simulink model "svpwm_inv_Motor_new_sent"  (R2022b)
settings: Solver=daessc  StartTime=0.0  StopTime=0.62  MaxStep=2.5e-6  RelTol=1e-3
libraries: nesl_utility x37, fl_lib x34, ee_lib x21, spsMeanLib x9, simulink x6, slpidlib x4, mcbcontrolslib x3, simulink_extras x1
(part 2 of 2)

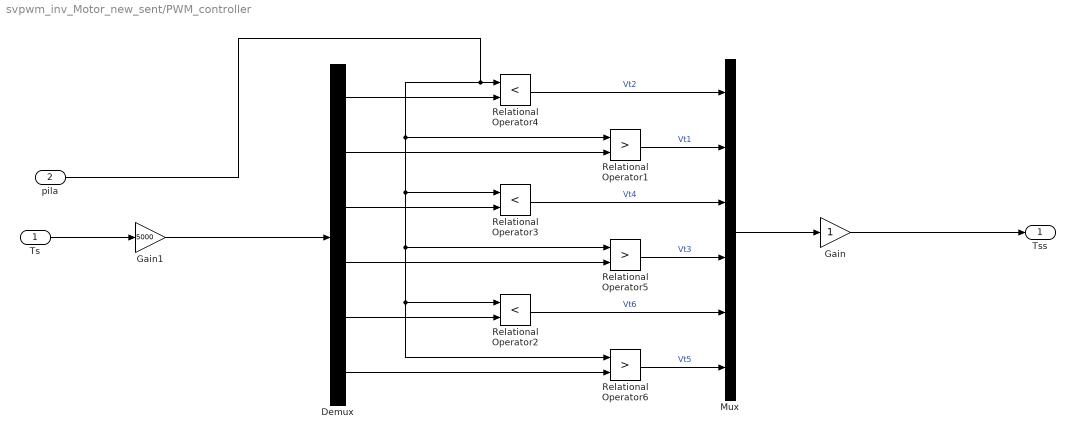
== system svpwm_inv_Motor_new_sent/PWM_controller ==
  Ts : Inport
  pila : Inport  Port=2
  Demux : Demux  Outputs=6
  Gain : Gain  ParamDataTypeStr=double
  Gain1 : Gain  Gain=5000
  Mux : Mux  Inputs=6
  Relational Operator1 : RelationalOperator  Operator=>  OutDataTypeStr=boolean  InputSameDT=off
  Relational Operator2 : RelationalOperator  Operator=<  OutDataTypeStr=boolean  InputSameDT=off
  Relational Operator3 : RelationalOperator  Operator=<  OutDataTypeStr=boolean  InputSameDT=off
  Relational Operator4 : RelationalOperator  Operator=<  OutDataTypeStr=boolean  InputSameDT=off
  Relational Operator5 : RelationalOperator  Operator=>  OutDataTypeStr=boolean  InputSameDT=off
  Relational Operator6 : RelationalOperator  Operator=>  OutDataTypeStr=boolean  InputSameDT=off
  Tss : Outport  VectorParamsAs1DForOutWhenUnconnected=off
  wires:
  Relational Operator4/1 -> Mux/1  "Vt2"
  Demux/3 -> Relational Operator3/2
  Demux/5 -> Relational Operator2/2
  Relational Operator3/1 -> Mux/3  "Vt4"
  Relational Operator2/1 -> Mux/5  "Vt6"
  Ts/1 -> Gain1/1
  pila/1 -> Relational Operator1/1, Relational Operator3/1, Relational Operator5/1, Relational Operator2/1, Relational Operator6/1, Relational Operator4/1
  Relational Operator1/1 -> Mux/2  "Vt1"
  Relational Operator5/1 -> Mux/4  "Vt3"
  Relational Operator6/1 -> Mux/6  "Vt5"
  Demux/2 -> Relational Operator1/2
  Demux/4 -> Relational Operator5/2
  Demux/6 -> Relational Operator6/2
  Demux/1 -> Relational Operator4/2
  Mux/1 -> Gain/1
  Gain/1 -> Tss/1
  Gain1/1 -> Demux/1

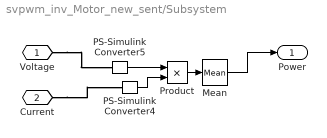
== system svpwm_inv_Motor_new_sent/Subsystem ==
  Mean : spsMeanLib/Mean  Freq=5000  Vinit=0  Ts=0
  PS-Simulink Converter4 : nesl_utility/PS-Simulink Converter  PhysicalDomain=network_engine_domain  SubClassName=ps_output  LeftPortType=input  RightPortType=output  PseudoPeriodic=off  Frequencies=[]  VectorFormat=inherit  Unit=inherit  AffineConversion=off
  PS-Simulink Converter5 : nesl_utility/PS-Simulink Converter  PhysicalDomain=network_engine_domain  SubClassName=ps_output  LeftPortType=input  RightPortType=output  PseudoPeriodic=off  Frequencies=[]  VectorFormat=inherit  Unit=inherit  AffineConversion=off
  Product : Product
  Voltage : PMIOPort  Side=Left
  Current : PMIOPort  Port=2  Side=Left
  Power : Outport
  wires:
  Product/1 -> Mean/1
  PS-Simulink Converter5/1 -> Product/1
  PS-Simulink Converter4/1 -> Product/2
  Mean/1 -> Power/1
  connections:
  Current/RConn1 -- PS-Simulink Converter4/LConn1
  Voltage/RConn1 -- PS-Simulink Converter5/LConn1

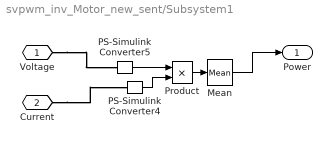
== system svpwm_inv_Motor_new_sent/Subsystem1 ==
  Mean : spsMeanLib/Mean  Freq=5000  Vinit=0  Ts=0
  PS-Simulink Converter4 : nesl_utility/PS-Simulink Converter  PhysicalDomain=network_engine_domain  SubClassName=ps_output  LeftPortType=input  RightPortType=output  PseudoPeriodic=off  Frequencies=[]  VectorFormat=inherit  Unit=inherit  AffineConversion=off
  PS-Simulink Converter5 : nesl_utility/PS-Simulink Converter  PhysicalDomain=network_engine_domain  SubClassName=ps_output  LeftPortType=input  RightPortType=output  PseudoPeriodic=off  Frequencies=[]  VectorFormat=inherit  Unit=inherit  AffineConversion=off
  Product : Product
  Voltage : PMIOPort  Side=Left
  Current : PMIOPort  Port=2  Side=Left
  Power : Outport
  wires:
  Mean/1 -> Power/1
  PS-Simulink Converter4/1 -> Product/2
  PS-Simulink Converter5/1 -> Product/1
  Product/1 -> Mean/1
  connections:
  Voltage/RConn1 -- PS-Simulink Converter5/LConn1
  Current/RConn1 -- PS-Simulink Converter4/LConn1

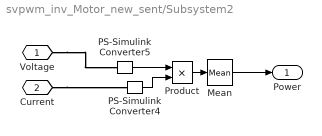
== system svpwm_inv_Motor_new_sent/Subsystem2 ==
  Mean : spsMeanLib/Mean  Freq=5000  Vinit=0  Ts=0
  PS-Simulink Converter4 : nesl_utility/PS-Simulink Converter  PhysicalDomain=network_engine_domain  SubClassName=ps_output  LeftPortType=input  RightPortType=output  PseudoPeriodic=off  Frequencies=[]  VectorFormat=inherit  Unit=inherit  AffineConversion=off
  PS-Simulink Converter5 : nesl_utility/PS-Simulink Converter  PhysicalDomain=network_engine_domain  SubClassName=ps_output  LeftPortType=input  RightPortType=output  PseudoPeriodic=off  Frequencies=[]  VectorFormat=inherit  Unit=inherit  AffineConversion=off
  Product : Product
  Voltage : PMIOPort  Side=Left
  Current : PMIOPort  Port=2  Side=Left
  Power : Outport
  wires:
  Mean/1 -> Power/1
  PS-Simulink Converter4/1 -> Product/2
  PS-Simulink Converter5/1 -> Product/1
  Product/1 -> Mean/1
  connections:
  Voltage/RConn1 -- PS-Simulink Converter5/LConn1
  Current/RConn1 -- PS-Simulink Converter4/LConn1

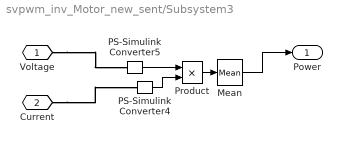
== system svpwm_inv_Motor_new_sent/Subsystem3 ==
  Mean : spsMeanLib/Mean  Freq=5000  Vinit=0  Ts=0
  PS-Simulink Converter4 : nesl_utility/PS-Simulink Converter  PhysicalDomain=network_engine_domain  SubClassName=ps_output  LeftPortType=input  RightPortType=output  PseudoPeriodic=off  Frequencies=[]  VectorFormat=inherit  Unit=inherit  AffineConversion=off
  PS-Simulink Converter5 : nesl_utility/PS-Simulink Converter  PhysicalDomain=network_engine_domain  SubClassName=ps_output  LeftPortType=input  RightPortType=output  PseudoPeriodic=off  Frequencies=[]  VectorFormat=inherit  Unit=inherit  AffineConversion=off
  Product : Product
  Voltage : PMIOPort  Side=Left
  Current : PMIOPort  Port=2  Side=Left
  Power : Outport
  wires:
  Product/1 -> Mean/1
  PS-Simulink Converter5/1 -> Product/1
  PS-Simulink Converter4/1 -> Product/2
  Mean/1 -> Power/1
  connections:
  Current/RConn1 -- PS-Simulink Converter4/LConn1
  Voltage/RConn1 -- PS-Simulink Converter5/LConn1

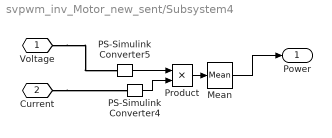
== system svpwm_inv_Motor_new_sent/Subsystem4 ==
  Mean : spsMeanLib/Mean  Freq=5000  Vinit=0  Ts=0
  PS-Simulink Converter4 : nesl_utility/PS-Simulink Converter  PhysicalDomain=network_engine_domain  SubClassName=ps_output  LeftPortType=input  RightPortType=output  PseudoPeriodic=off  Frequencies=[]  VectorFormat=inherit  Unit=inherit  AffineConversion=off
  PS-Simulink Converter5 : nesl_utility/PS-Simulink Converter  PhysicalDomain=network_engine_domain  SubClassName=ps_output  LeftPortType=input  RightPortType=output  PseudoPeriodic=off  Frequencies=[]  VectorFormat=inherit  Unit=inherit  AffineConversion=off
  Product : Product
  Voltage : PMIOPort  Side=Left
  Current : PMIOPort  Port=2  Side=Left
  Power : Outport
  wires:
  Mean/1 -> Power/1
  PS-Simulink Converter4/1 -> Product/2
  PS-Simulink Converter5/1 -> Product/1
  Product/1 -> Mean/1
  connections:
  Voltage/RConn1 -- PS-Simulink Converter5/LConn1
  Current/RConn1 -- PS-Simulink Converter4/LConn1

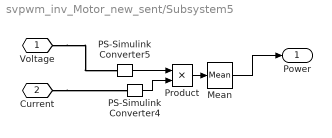
== system svpwm_inv_Motor_new_sent/Subsystem5 ==
  Mean : spsMeanLib/Mean  Freq=5000  Vinit=0  Ts=0
  PS-Simulink Converter4 : nesl_utility/PS-Simulink Converter  PhysicalDomain=network_engine_domain  SubClassName=ps_output  LeftPortType=input  RightPortType=output  PseudoPeriodic=off  Frequencies=[]  VectorFormat=inherit  Unit=inherit  AffineConversion=off
  PS-Simulink Converter5 : nesl_utility/PS-Simulink Converter  PhysicalDomain=network_engine_domain  SubClassName=ps_output  LeftPortType=input  RightPortType=output  PseudoPeriodic=off  Frequencies=[]  VectorFormat=inherit  Unit=inherit  AffineConversion=off
  Product : Product
  Voltage : PMIOPort  Side=Left
  Current : PMIOPort  Port=2  Side=Left
  Power : Outport
  wires:
  Product/1 -> Mean/1
  PS-Simulink Converter5/1 -> Product/1
  PS-Simulink Converter4/1 -> Product/2
  Mean/1 -> Power/1
  connections:
  Current/RConn1 -- PS-Simulink Converter4/LConn1
  Voltage/RConn1 -- PS-Simulink Converter5/LConn1

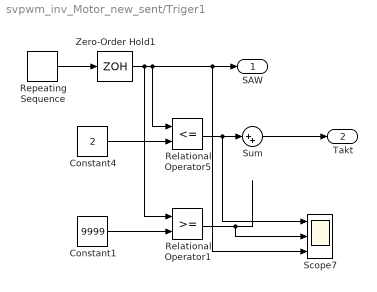
== system svpwm_inv_Motor_new_sent/Triger1 ==
  Constant1 : Constant  Value=9999
  Constant4 : Constant  Value=2
  Relational Operator1 : RelationalOperator  OutDataTypeStr=boolean  InputSameDT=off
  Relational Operator5 : RelationalOperator  Operator=<=  OutDataTypeStr=boolean  InputSameDT=off
  Repeating Sequence : simulink/Sources/Repeating Sequence  rep_seq_t=[0 40e-6 80e-6]  rep_seq_y=[0 5000 0]
  Scope7 : Scope  NumInputPorts=3
  Sum : Sum  Inputs=|++
  Zero-Order Hold1 : ZeroOrderHold  SampleTime=2.5e-7
  SAW : Outport  VectorParamsAs1DForOutWhenUnconnected=off
  Takt : Outport  Port=2  VectorParamsAs1DForOutWhenUnconnected=off
  wires:
  Zero-Order Hold1/1 -> Relational Operator1/1, Relational Operator5/1, Scope7/3, SAW/1
  Repeating Sequence/1 -> Zero-Order Hold1/1
  Constant4/1 -> Relational Operator5/2
  Sum/1 -> Takt/1
  Constant1/1 -> Relational Operator1/2
  Relational Operator5/1 -> Scope7/1, Sum/1
  Relational Operator1/1 -> Scope7/2

== matlab function svpwm_inv_Motor_new_sent/SVPWM ==
  data: vrefa input; vphase input; VDC input; IA input; IB input; Ts output
  events: trigger input RISING_EDGE_EVENT
%function [Ts1,Ts2,Ts3,Ts4,Ts5,Ts6] = fcn(vrefa,vphase,VDC,IA,IB)
function Ts   = fcn(vrefa,vphase,VDC,IA,IB)
%время 1/2 ШИМ периода
dt=80e-6;


%алгоритм формирования векторной ШИМ  мертвым веменем dead [мкс]
dead=0.75;
dead=dead/(dt*1e6);
a=vphase;
v2=vrefa;
if a>=0 && a<pi/3 
    n=1;
elseif  a>=pi/3 && a<2*pi/3 
    n=2;
elseif  a>=2*pi/3 && a<pi 
    n=3;
elseif  a>=pi && a<4*pi/3 
    n=4;
elseif  a>=4*pi/3 && a<5*pi/3 
    n=5;
else n=6;

end

a_cor=a-(n-1)*pi/3;

T1 = (v2/VDC)*sin(pi/3-a_cor)/sin(pi/3);
T2 = (v2/VDC)*sin(a_cor)/sin(pi/3);
T0=1-T1-T2;
Ta1=0; Ta3=0; Ta5=0; 
switch n
    case 1
        
        Ta1=T1+T2+T0/2;
        
        Ta3=T2+T0/2;
       
        Ta5=T0/2;
       
    case 2
        
        Ta1=T1+T0/2;
        
        Ta3=T1+T2+T0/2;
    
        Ta5=T0/2;       
        
    case 3
        
        Ta1=T0/2;
       
        Ta3=T1+T2+T0/2;
       
        Ta5=T2+T0/2;    
        
    case 4
        
        Ta1=T0/2;
       
        Ta3=T1+T0/2;
       
        Ta5=T1+T2+T0/2;   
       
    case 5
        
        Ta1=T2+T0/2;
        
        Ta3=T0/2;
        
        Ta5=T1+T2+T0/2;     
        
    case 6
        
        Ta1=T1+T2+T0/2;
        
        Ta3=T0/2;
     
        Ta5=T1+T0/2;    
        
end

if (Ta1 >0.95)
    Ta1 = 0.95;
elseif (Ta1 < 0.05)
        Ta1 = 0.05;
end

if (Ta3 >0.95)
    Ta3 = 0.95;
elseif (Ta3 < 0.05)
        Ta3 = 0.05;
end

if (Ta5 >0.95)
    Ta5 = 0.95;
elseif (Ta5 < 0.05)
        Ta5 = 0.05;
end


Ts1=(Ta1)-dead/2; 
Ts3=(Ta3)-dead/2; 
Ts5=(Ta5)-dead/2;
Ts2=(Ta1)+dead/2; 
Ts4=(Ta3)+dead/2; 
Ts6=(Ta5)+dead/2;


if (IA>0) 
    Ts1=Ts1+dead/2;
    Ts2=Ts2+dead/2;
else
    Ts1=Ts1-dead/2;
    Ts2=Ts2-dead/2;           
end
if (IB>0) 
    Ts3=Ts3+dead/2;
    Ts4=Ts4+dead/2;
else
    Ts3=Ts3-dead/2;
    Ts4=Ts4-dead/2; 
end  
if ((-IA-IB)>0) 
    Ts5=Ts5+dead/2;
    Ts6=Ts6+dead/2;
else
    Ts5=Ts5-dead/2;
    Ts6=Ts6-dead/2;           
end

Ts = [Ts1,Ts2,Ts3,Ts4,Ts5,Ts6];
return;

== matlab function svpwm_inv_Motor_new_sent/MATLAB Function ==
  data: u input; y output
function y = fcn(u)
if (u ~= 0)
    y = u;
else
    y = 1e-6;
end
